simulink model "double_pendulum_minimal_rightversion"  (R2024b)
settings: Solver=ode15s  StartTime=0.0  StopTime=10.0  RelTol=1e-3
settings Model: Creator=yang  LastModifiedBy=yang

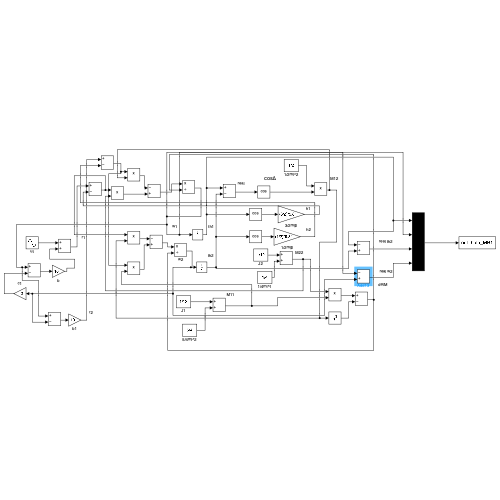
[thumbnail: Simulink's stored preview of the top-level diagram]
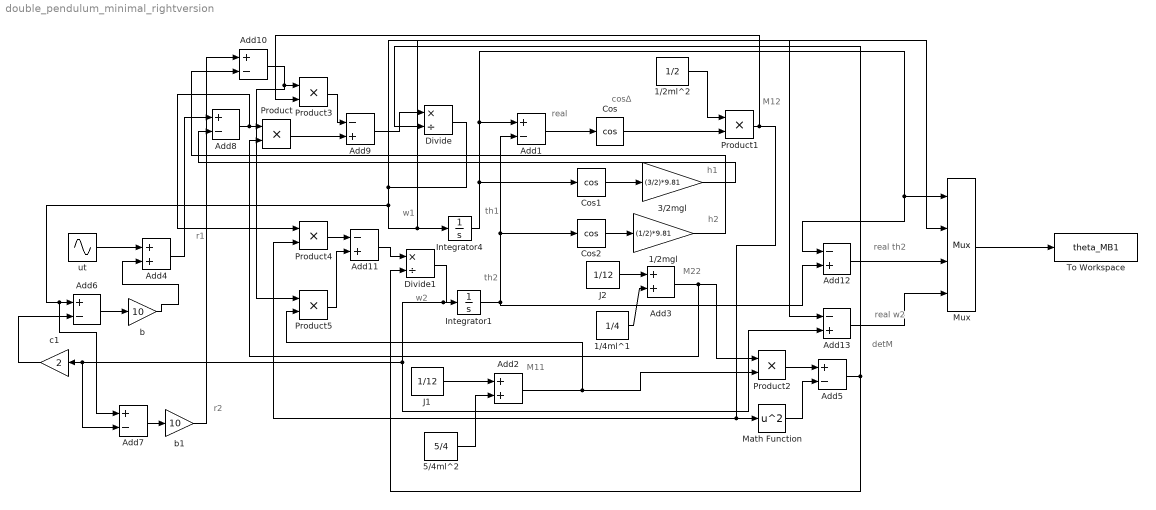
== system double_pendulum_minimal_rightversion ==
  note: real th2
  note: r2
  note: r1
  note: h2
  note: h1
  note: detM
  note: M22
  note: M12
  note: M11
  note: cosΔ
  note: real
  note: w2
  note: w1
  note: th2
  note: th1
  note: real w2
  1/2mgl : Gain  Gain=(1/2)*9.81
  1/2ml^2 : Constant  Value=1/2
  1/4ml^1 : Constant  Value=1/4
  3/2mgl : Gain  Gain=(3/2)*9.81
  5/4ml^2 : Constant  Value=5/4
  Add{1,5..8,10} (6 alike) : Sum  Inputs=+-
  Add{9,11..13} (4 alike) : Sum  Inputs=-+
  Add2 : Sum
  Add3 : Sum
  Add4 : Sum
  Cos : Trigonometry  Operator=cos
  Cos1 : Trigonometry  Operator=cos
  Cos2 : Trigonometry  Operator=cos
  Divide : Product  Inputs=*/
  Divide1 : Product  Inputs=*/
  Integrator1 : Integrator
  Integrator4 : Integrator
  J1 : Constant  Value=1/12
  J2 : Constant  Value=1/12
  Math Function : Math  Operator=square
  Mux : Mux
  Product{,1..5} (6 alike) : Product
  To Workspace : ToWorkspace  VariableName=theta_MB1  SaveFormat=Timeseries  SampleTime=-1
  b : Gain  Gain=10
  b1 : Gain  Gain=10
  c1 : Gain  Gain=2
  ut : Sin  Amplitude=5  Frequency=5  SampleTime=0
  wires:
  Mux/1 -> To Workspace/1
  Divide/1 -> Mux/2, Integrator4/1, Add7/1, Add6/1, Add13/1
  Divide1/1 -> Add13/2, Add7/2, c1/1, Integrator1/1
  Integrator4/1 -> Add12/1, Mux/1, Add1/1, Cos1/1
  Integrator1/1 -> Add1/2, Cos2/1, Add12/2
  Add1/1 -> Cos/1
  J1/1 -> Add2/1
  5/4ml^2/1 -> Add2/2
  Add2/1 -> Product5/2, Product2/2
  Cos/1 -> Product1/2
  1/2ml^2/1 -> Product1/1
  Product1/1 -> Product4/2, Math Function/1, Product3/2
  Add3/1 -> Product/2, Product2/1
  J2/1 -> Add3/1
  1/4ml^1/1 -> Add3/2
  Product2/1 -> Add5/1
  Math Function/1 -> Add5/2
  Cos1/1 -> 3/2mgl/1
  3/2mgl/1 -> Add8/2
  Cos2/1 -> 1/2mgl/1
  1/2mgl/1 -> Add10/2
  ut/1 -> Add4/1
  Add6/1 -> b/1
  b/1 -> Add4/2
  c1/1 -> Add6/2
  Add7/1 -> b1/1
  b1/1 -> Add10/1
  Add4/1 -> Add8/1
  Add8/1 -> Product4/1, Product/1
  Product/1 -> Add9/2
  Add10/1 -> Product5/1, Product3/1
  Product3/1 -> Add9/1
  Add9/1 -> Divide/1
  Add5/1 -> Divide/2, Divide1/2
  Product4/1 -> Add11/1
  Product5/1 -> Add11/2
  Add11/1 -> Divide1/1
  Add12/1 -> Mux/3
  Add13/1 -> Mux/4
